simulink model "ESE4481MController"  (R2024a)
settings: Solver=VariableStepAuto  StartTime=0.0  StopTime=10.0  RelTol=1e-3
undefined symbols (not defined in the file): g, Jy, Kpn, Kq, Ktheta, Ku, Pnc
settings Model: Creator=achic  LastModifiedBy=achic

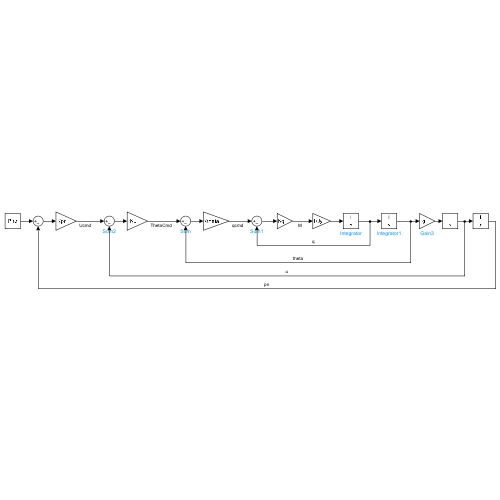
[thumbnail: Simulink's stored preview of the top-level diagram]
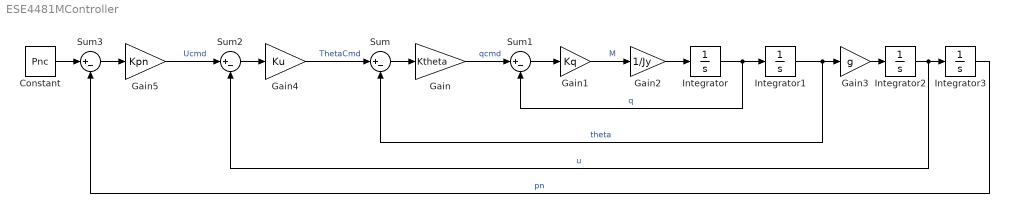
== system ESE4481MController ==
  Constant : Constant  Value=Pnc
  Gain : Gain  Gain=Ktheta
  Gain1 : Gain  Gain=Kq
  Gain2 : Gain  Gain=1/Jy
  Gain3 : Gain  Gain=g
  Gain4 : Gain  Gain=Ku
  Gain5 : Gain  Gain=Kpn
  Integrator{,1..3} (4 alike) : Integrator
  Sum{,1..3} (4 alike) : Sum  Inputs=|+-
  wires:
  Gain5/1 -> Sum2/1  "Ucmd"
  Gain2/1 -> Integrator/1
  Gain/1 -> Sum1/1  "qcmd"
  Integrator1/1 -> Gain3/1, Sum/2  "theta"
  Integrator3/1 -> Sum3/2  "pn"
  Gain1/1 -> Gain2/1  "M"
  Gain3/1 -> Integrator2/1
  Gain4/1 -> Sum/1  "ThetaCmd"
  Integrator2/1 -> Integrator3/1, Sum2/2  "u"
  Constant/1 -> Sum3/1
  Integrator/1 -> Integrator1/1, Sum1/2  "q"
  Sum1/1 -> Gain1/1
  Sum/1 -> Gain/1
  Sum2/1 -> Gain4/1
  Sum3/1 -> Gain5/1
